simulink model "lab2_symulacja"  (R2022a)
settings: Solver=VariableStepAuto  StartTime=0.0  StopTime=40.0  MaxStep=0.01  RelTol=1e-3
values from neighbouring files (symbols this model uses):
  k = 2    [lab2.m]
  omega = 1/16    (= 0.0625)    [lab2.m]
  T_stala = 6    [lab2.m]
settings Model: Creator=rober  LastModifiedBy=rober

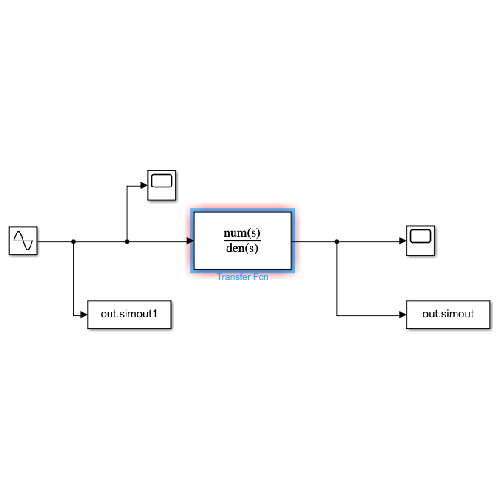
[thumbnail: Simulink's stored preview of the top-level diagram]
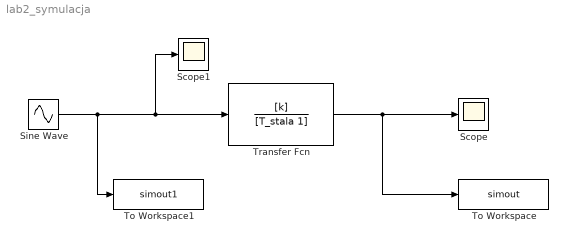
== system lab2_symulacja ==
  Scope : Scope
  Scope1 : Scope
  Sine Wave : Sin  Frequency=omega  SampleTime=0
  To Workspace : ToWorkspace  VariableName=simout  SampleTime=-1
  To Workspace1 : ToWorkspace  VariableName=simout1  SampleTime=-1
  Transfer Fcn : TransferFcn  Numerator=[k]  Denominator=[T_stala 1]
  wires:
  Sine Wave/1 -> To Workspace1/1, Scope1/1, Transfer Fcn/1
  Transfer Fcn/1 -> To Workspace/1, Scope/1
